simulink model "myCsystem"  (R2018a)
settings: Solver=VariableStepAuto  StartTime=0.0  StopTime=59  RelTol=1e-3
libraries: commblkcod2 x2, commchan3 x1, commsink2 x1, commrandsrc3 x1
settings Model: Creator=lenovo  LastModifiedBy=lenovo

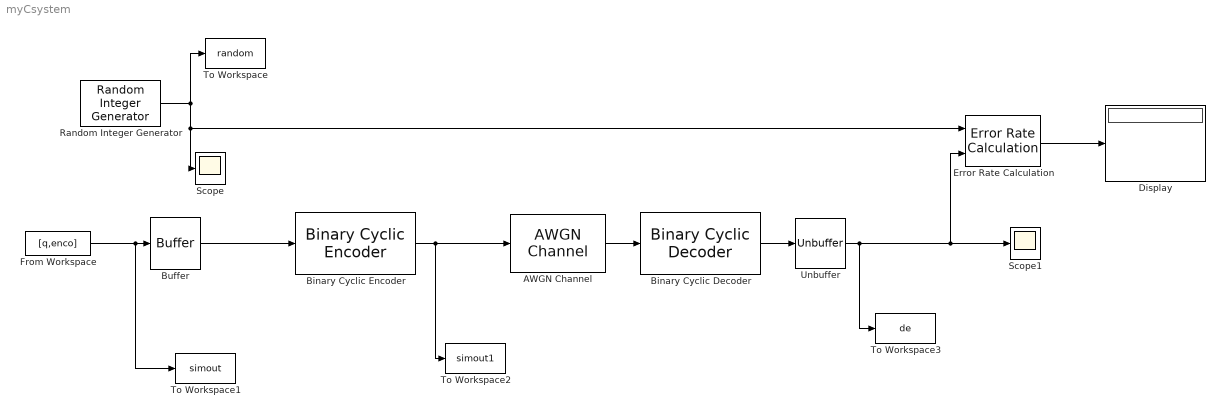
== system myCsystem ==
  AWGN Channel : commchan3/AWGN Channel  InputProcessing=Columns as channels (frame based)  seed=67  noiseMode="Signal to noise ratio  (Eb/No)"  EbNodB=10  EsNodB=10  SNRdB=10  bitsPerSym=1  Ps=1  Tsym=1  variance=1
  Binary Cyclic Decoder : commblkcod2/Binary Cyclic Decoder  n=7  p=4
      settings: SourceProductName=Communications System Toolbox  SourceProductBaseCode=CM
  Binary Cyclic Encoder : commblkcod2/Binary Cyclic Encoder  n=7  p=4
      settings: SourceProductName=Communications System Toolbox  SourceProductBaseCode=CM
  Buffer : Buffer  N=4  OutputFrames=off
  Display : Display
  Error Rate Calculation : commsink2/Error Rate Calculation  N=0  st_delay=0  cp_mode=Entire frame  subframe=[]  PMode=Port  WsName=ErrorVec  RsMode2=off  stop=off  numErr=100  maxBits=1e6
  From Workspace : FromWorkspace  VariableName=[q,enco]
  Random Integer Generator : commrandsrc3/Random Integer Generator  SetSize=2  SeedSource=Auto  Seed=0  SampleTime=1  SamplesPerFrame=1  OutputDataType=double  SimulateUsing=Interpreted execution
  Scope : Scope
  Scope1 : Scope
  To Workspace : ToWorkspace  VariableName=random  SampleTime=-1
      settings: Save2DSignal=2-D array (concatenate along first dimension)
  To Workspace1 : ToWorkspace  VariableName=simout  SampleTime=-1
      settings: Save2DSignal=2-D array (concatenate along first dimension)
  To Workspace2 : ToWorkspace  VariableName=simout1  SampleTime=-1
      settings: Save2DSignal=2-D array (concatenate along first dimension)
  To Workspace3 : ToWorkspace  VariableName=de  SampleTime=-1
      settings: Save2DSignal=2-D array (concatenate along first dimension)
  Unbuffer : Unbuffer
  wires:
  Binary Cyclic Encoder/1 -> To Workspace2/1, AWGN Channel/1
  Random Integer Generator/1 -> Error Rate Calculation/1, Scope/1, To Workspace/1
  From Workspace/1 -> To Workspace1/1, Buffer/1
  AWGN Channel/1 -> Binary Cyclic Decoder/1
  Buffer/1 -> Binary Cyclic Encoder/1
  Binary Cyclic Decoder/1 -> Unbuffer/1
  Unbuffer/1 -> Error Rate Calculation/2, Scope1/1, To Workspace3/1
  Error Rate Calculation/1 -> Display/1
